simulink model "modeleSIGUI"  (R2020b)
settings: Solver=VariableStepAuto  StartTime=0.0  StopTime=100  RelTol=1e-3
values from neighbouring files (symbols this model uses):
  D = dec2bin(int32(decMatrix(:, 3)*100), bits)    [BinPopGUI.m]    (also in DecPopGUI.m = bin2dec(binMatrix(:, 2*n/3+1:n))/100; PIDOptimFuncGUI.m = PID(3); StartPopGUI.m = randi(range, [population, 1]))
  I = dec2bin(int32(decMatrix(:, 2)*100), bits)    [BinPopGUI.m]    (also in DecPopGUI.m = bin2dec(binMatrix(:, n/3+1:2*n/3))/100; PIDOptimFuncGUI.m = PID(2); StartPopGUI.m = randi(range, [population, 1]))
  k = model(1)    [PIDOptimFuncGUI.m]    (also in Pairing2GUI.m = randi(j))
  P = dec2bin(int32(decMatrix(:, 1)*100), bits)    [BinPopGUI.m]    (also in DecPopGUI.m = bin2dec(binMatrix(:, 1:n/3))/100; PIDOptimFuncGUI.m = PID(1); StartPopGUI.m = randi(range, [population, 1]))
  T1 = model(2)    [PIDOptimFuncGUI.m]
  T2 = model(3)    [PIDOptimFuncGUI.m]
  tau = model(4)    [PIDOptimFuncGUI.m]
libraries: pid_lib x1
settings Model: Creator=jaron  LastModifiedBy=jaron

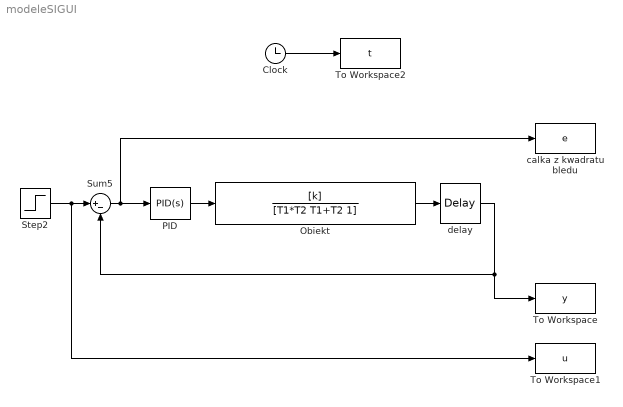
== system modeleSIGUI ==
  Clock : Clock
  Obiekt : TransferFcn  Numerator=[k]  Denominator=[T1*T2 T1+T2 1]
  PID : pid_lib/PID Controller  Controller=PID  Form=Parallel  TimeDomain=Continuous-time  UseExternalTs=off  SampleTime=-1  IntegratorMethod=Forward Euler  FilterMethod=Forward Euler  ControllerParametersSource=internal  P=P  I=I  D=D  UseFilter=on  N=100  TunerSelectOption=Transfer Function Based (PID Tuner App)  InitialConditionSource=internal  InitialConditionForIntegrator=0  InitialConditionForFilter=0  DifferentiatorICPrevScaledInput=0  ExternalReset=none  TrackingMode=off  Kt=1  LimitOutput=off  SatLimitsSource=internal  UpperSaturationLimit=inf  LowerSaturationLimit=-inf  LinearizeAsGain=on  AntiWindupMode=none  Kb=1  POutMin=[]  POutMax=[]  IOutMin=[]  IOutMax=[]  DOutMin=[]  DOutMax=[]  NOutMin=[]  NOutMax=[]  SumOutMin=[]  SumOutMax=[]  SaturationOutMin=[]  SaturationOutMax=[]  PParamMin=[]  PParamMax=[]  IParamMin=[]  IParamMax=[]  DParamMin=[]  DParamMax=[]  NParamMin=[]  NParamMax=[]  KbParamMin=[]  KbParamMax=[]  KtParamMin=[]  KtParamMax=[]  KbOutMin=[]  KbOutMax=[]  KtOutMin=[]  KtOutMax=[]  IntegratorOutMin=[]  IntegratorOutMax=[]  FilterOutMin=[]  FilterOutMax=[]  SumI1OutMin=[]  SumI1OutMax=[]  SumI2OutMin=[]  SumI2OutMax=[]  SumI3OutMin=[]  SumI3OutMax=[]  SumI4OutMin=[]  SumI4OutMax=[]  SumDOutMin=[]  SumDOutMax=[]  DifferentiatorOutMin=[]  DifferentiatorOutMax=[]  FilterDiffOutCoefMin=[]  FilterDiffOutCoefMax=[]  ReciprocalOutMin=[]  ReciprocalOutMax=[]  SumDenOutMin=[]  SumDenOutMax=[]  SumNumOutMin=[]  SumNumOutMax=[]  DivideOutMin=[]  DivideOutMax=[]  UdiffTsProdOutMin=[]  UdiffTsProdOutMax=[]  NTsProdOutMin=[]  NTsProdOutMax=[]  UintegralTsProdOutMin=[]  UintegralTsProdOutMax=[]  UngainTsProdOutMin=[]  UngainTsProdOutMax=[]  IntegratorContinuousStateAttributes=''  IntegratorStateMustResolveToSignalObject=off  IntegratorRTWStateStorageClass=Auto  FilterContinuousStateAttributes=''  FilterStateMustResolveToSignalObject=off  FilterRTWStateStorageClass=Auto  ParallelPVariant=InternalParameters  IdealPVariant=Disabled  IVariant=InternalParameters  DVariant=InternalParameters  IntegratorVariant=Continuous  SatVariant=Disabled  AWVariant=Passthrough  PCopyVariant=Disabled  TRVariant=Disabled  FdbkBlocksVariant=Forward  IdealPFdbkVariant=Disabled  SatFdbkVariant=Disabled  DerivativeFilterVariant=ContFilter  NVariant=InternalParameters  NCopyVariant=Disabled  FilterICVariant=InternalICsFilter  IntegratorICVariant=InternalICs  ExternalResetVariant=Disabled  TRSumVariant=Passthrough  SumFdbkVariant=Disabled  SumVariant=Sum_PID  TsampFilterVariant=InternalTs  TsampNgainVariant=Passthrough  TsampIntegralVariant=Passthrough  ExternalSaturationOutDataTypeStr=Inherit: Same as second input
  Step2 : Step  Time=0  SampleTime=0
  Sum5 : Sum  Inputs=|+-
  To Workspace : ToWorkspace  VariableName=y  SampleTime=0.1
  To Workspace1 : ToWorkspace  VariableName=u  SampleTime=0.1
  To Workspace2 : ToWorkspace  VariableName=t  SampleTime=0.1
  calka z kwadratu bledu : ToWorkspace  VariableName=e  SampleTime=0.1
  delay : TransportDelay  DelayTime=tau
  wires:
  Obiekt/1 -> delay/1
  PID/1 -> Obiekt/1
  Step2/1 -> Sum5/1, To Workspace1/1
  Clock/1 -> To Workspace2/1
  delay/1 -> Sum5/2, To Workspace/1
  Sum5/1 -> PID/1, calka z kwadratu bledu/1
